simulink model "Mooventure2016_Rev5"  (Simulink 7.7)
settings: Solver=FixedStepDiscrete  StartTime=0.0  StopTime=10  RelTol=1e-3
PreLoadFcn:
  | try, eval([bdroot '_setup']); catch, eval('model_setup', ''); end
InitFcn:
  | try, eval([bdroot '_setup']); catch, eval('model_setup', ''); end
undefined symbols (not defined in the file): ECM, H1, motohawk_build_version, motohawk_trunc_name, motohawk_vardec_config_group, motohawk_vardec_path, xD
libraries: MotoHawk_lib x976, motohawk_control_primitives_lib x41, simulink x27, motohawk_annotations_lib x3
(part 9 of 16)

== system Mooventure2016_Rev5/Foreground/Control/Hybrid Control Code/EcoMode ==
  note: This is brake pedal regen mode
  Inputs : Inport
  InReverse : Inport  Port=2
  Action Port : ActionPort  ActionType=case
  Brake Pedal Scaling : Stateflow chart  TreatAsAtomicUnit=on
  Bus Selector : BusSelector  OutputSignals=Driver Inputs.Throttle_Position (signal 5),Driver Inputs.Brake_Position (signal 2)
  Bus Selector1 : BusSelector  OutputSignals=IPT.ID 260 IPT Status 2.IPT_MotorSpeed
  Chart : Stateflow chart  TreatAsAtomicUnit=on
  Constant : Constant
  Data Type Conversion : DataTypeConversion  OutDataTypeStr=double
  Data Type Conversion1 : DataTypeConversion  OutDataTypeStr=double
  Gas Pedal Scaling : Stateflow chart  TreatAsAtomicUnit=on
  Product : Product  RndMeth=Zero
  Product1 : Product  RndMeth=Zero
  Product2 : Product  RndMeth=Zero
  Sum : Sum
  motohawk_calibration : MotoHawk_lib/Calibration & Probing Blocks/motohawk_calibration  nam='accelStart_Pedal_ecoMode'  val=.02  storage=Calibration  show_more=off  name_source=Use Parameter  data_type=Inherit from 'Default Value'  read_level=1  write_level=1  ovr_cals=on  view_as=Number  enum_struct={'Disabled', 'Enabled'}  vector_style=Wide Row  use_help_units=off  help=''  units=''  use_header_enum=off  row_header_enum={}  col_header_enum={}  use_min_max=off  min_val=-inf  max_val=inf  use_precision=off  precision=''  gain=1  offset=0  exp=1  use_mototune_group=off  mototune_group=motohawk_vardec_path(gcb)
  motohawk_calibration1 : MotoHawk_lib/Calibration & Probing Blocks/motohawk_calibration  nam='brakeStart_Pedal_ecoMode'  val=.02  storage=Calibration  show_more=off  name_source=Use Parameter  data_type=Inherit from 'Default Value'  read_level=1  write_level=1  ovr_cals=on  view_as=Number  enum_struct={'Disabled', 'Enabled'}  vector_style=Wide Row  use_help_units=off  help=''  units=''  use_header_enum=off  row_header_enum={}  col_header_enum={}  use_min_max=off  min_val=-inf  max_val=inf  use_precision=off  precision=''  gain=1  offset=0  exp=1  use_mototune_group=off  mototune_group=motohawk_vardec_path(gcb)
  motohawk_calibration2 : MotoHawk_lib/Calibration & Probing Blocks/motohawk_calibration  nam='brakeEnd_Pedal_ecoMode'  val=.01  storage=Calibration  show_more=off  name_source=Use Parameter  data_type=Inherit from 'Default Value'  read_level=1  write_level=1  ovr_cals=on  view_as=Number  enum_struct={'Disabled', 'Enabled'}  vector_style=Wide Row  use_help_units=off  help=''  units=''  use_header_enum=off  row_header_enum={}  col_header_enum={}  use_min_max=off  min_val=-inf  max_val=inf  use_precision=off  precision=''  gain=1  offset=0  exp=1  use_mototune_group=off  mototune_group=motohawk_vardec_path(gcb)
  motohawk_calibration3 : MotoHawk_lib/Calibration & Probing Blocks/motohawk_calibration  nam='regenStart_Speed_ecoMode'  val=2  storage=Calibration  show_more=off  name_source=Use Parameter  data_type=Inherit from 'Default Value'  read_level=1  write_level=1  ovr_cals=on  view_as=Number  enum_struct={'Disabled', 'Enabled'}  vector_style=Wide Row  use_help_units=off  help=''  units=''  use_header_enum=off  row_header_enum={}  col_header_enum={}  use_min_max=off  min_val=-inf  max_val=inf  use_precision=off  precision=''  gain=1  offset=0  exp=1  use_mototune_group=off  mototune_group=motohawk_vardec_path(gcb)
  motohawk_calibration4 : MotoHawk_lib/Calibration & Probing Blocks/motohawk_calibration  nam='accelEnd_Pedal_ecoMode'  val=.01  storage=Calibration  show_more=off  name_source=Use Parameter  data_type=Inherit from 'Default Value'  read_level=1  write_level=1  ovr_cals=on  view_as=Number  enum_struct={'Disabled', 'Enabled'}  vector_style=Wide Row  use_help_units=off  help=''  units=''  use_header_enum=off  row_header_enum={}  col_header_enum={}  use_min_max=off  min_val=-inf  max_val=inf  use_precision=off  precision=''  gain=1  offset=0  exp=1  use_mototune_group=off  mototune_group=motohawk_vardec_path(gcb)
  motohawk_calibration5 : MotoHawk_lib/Calibration & Probing Blocks/motohawk_calibration  nam='regenEnd_Speed_ecoMode'  val=0.75  storage=Calibration  show_more=off  name_source=Use Parameter  data_type=Inherit from 'Default Value'  read_level=1  write_level=1  ovr_cals=on  view_as=Number  enum_struct={'Disabled', 'Enabled'}  vector_style=Wide Row  use_help_units=off  help=''  units=''  use_header_enum=off  row_header_enum={}  col_header_enum={}  use_min_max=off  min_val=-inf  max_val=inf  use_precision=off  precision=''  gain=1  offset=0  exp=1  use_mototune_group=off  mototune_group=motohawk_vardec_path(gcb)
  motohawk_calibration6 : MotoHawk_lib/Calibration & Probing Blocks/motohawk_calibration  nam='dragTorque_ecoMode'  val=.09  storage=Calibration  show_more=off  name_source=Use Parameter  data_type=Inherit from 'Default Value'  read_level=1  write_level=1  ovr_cals=on  view_as=Number  enum_struct={'Disabled', 'Enabled'}  vector_style=Wide Row  use_help_units=off  help=''  units=''  use_header_enum=off  row_header_enum={}  col_header_enum={}  use_min_max=off  min_val=-inf  max_val=inf  use_precision=off  precision=''  gain=1  offset=0  exp=1  use_mototune_group=off  mototune_group=motohawk_vardec_path(gcb)
  motohawk_calibration7 : MotoHawk_lib/Calibration & Probing Blocks/motohawk_calibration  nam='RPM_to_Wheel_Speed_Multiplier_ecoMode'  val=0.01001896  storage=Calibration  show_more=off  name_source=Use Parameter  data_type=Inherit from 'Default Value'  read_level=1  write_level=1  ovr_cals=on  view_as=Number  enum_struct={'Disabled', 'Enabled'}  vector_style=Wide Row  use_help_units=off  help=''  units=''  use_header_enum=off  row_header_enum={}  col_header_enum={}  use_min_max=off  min_val=-inf  max_val=inf  use_precision=off  precision=''  gain=1  offset=0  exp=1  use_mototune_group=off  mototune_group=motohawk_vardec_path(gcb)
  motohawk_calibration8 : MotoHawk_lib/Calibration & Probing Blocks/motohawk_calibration  nam='driveMaxTorque_ecoMode'  val=1600  storage=Calibration  show_more=off  name_source=Use Parameter  data_type=Inherit from 'Default Value'  read_level=1  write_level=1  ovr_cals=on  view_as=Number  enum_struct={'Disabled', 'Enabled'}  vector_style=Wide Row  use_help_units=off  help=''  units=''  use_header_enum=off  row_header_enum={}  col_header_enum={}  use_min_max=off  min_val=-inf  max_val=inf  use_precision=off  precision=''  gain=1  offset=0  exp=1  use_mototune_group=off  mototune_group=motohawk_vardec_path(gcb)
  motohawk_calibration9 : MotoHawk_lib/Calibration & Probing Blocks/motohawk_calibration  nam='regenMaxTorque_ecoMode'  val=-1500  storage=Calibration  show_more=off  name_source=Use Parameter  data_type=Inherit from 'Default Value'  read_level=1  write_level=1  ovr_cals=on  view_as=Number  enum_struct={'Disabled', 'Enabled'}  vector_style=Wide Row  use_help_units=off  help=''  units=''  use_header_enum=off  row_header_enum={}  col_header_enum={}  use_min_max=off  min_val=-inf  max_val=inf  use_precision=off  precision=''  gain=1  offset=0  exp=1  use_mototune_group=off  mototune_group=motohawk_vardec_path(gcb)
  motohawk_interpolation_1d : MotoHawk_lib/Lookup Tables/motohawk_interpolation_1d  nam='EcoMode_Accel_Map'  table_data=[0:0.05:1]  show_more=on  data_type=double  storage=NonAdaptive  read_level=1  write_level=1  ovr_cals=on  use_help=off  help=''  units=''  use_min_max=off  min_val=0  max_val=1  use_precision=off  precision='1.2'  gain=1  offset=0  exp=1  use_links=on  prelookup_block='EcoMode_Accel'  output_name=''  use_mototune_group=off  mototune_group=motohawk_vardec_path(gcb)
  motohawk_interpolation_1d1 : MotoHawk_lib/Lookup Tables/motohawk_interpolation_1d  nam='EcoMode_Brake_Map'  table_data=[0:0.1:1,1,1,1,1,1,1,1,1,1,1]  show_more=on  data_type=double  storage=NonAdaptive  read_level=1  write_level=1  ovr_cals=on  use_help=off  help=''  units=''  use_min_max=off  min_val=0  max_val=1  use_precision=off  precision='1.2'  gain=1  offset=0  exp=1  use_links=on  prelookup_block='EcoMode_Brake'  output_name=''  use_mototune_group=off  mototune_group=motohawk_vardec_path(gcb)
  motohawk_prelookup : MotoHawk_lib/Lookup Tables/motohawk_prelookup  nam='EcoMode_Accel'  breakpoint_data=[0:0.05:1]  show_more=on  data_type=double  storage=Constant  read_level=1  write_level=1  ovr_cals=on  use_help=off  help=''  units=''  use_min_max=off  min_val=-inf  max_val=inf  use_precision=off  precision=''  gain=1  offset=0  exp=1  use_links=off  input_name=''  use_mototune_group=off  mototune_group=motohawk_vardec_path(gcb)
  motohawk_prelookup1 : MotoHawk_lib/Lookup Tables/motohawk_prelookup  nam='EcoMode_Brake'  breakpoint_data=[0:0.05:1]  show_more=on  data_type=double  storage=Constant  read_level=1  write_level=1  ovr_cals=on  use_help=off  help=''  units=''  use_min_max=off  min_val=-inf  max_val=inf  use_precision=off  precision=''  gain=1  offset=0  exp=1  use_links=off  input_name=''  use_mototune_group=off  mototune_group=motohawk_vardec_path(gcb)
  motohawk_probe : MotoHawk_lib/Calibration & Probing Blocks/motohawk_probe  nam='Gas_Pedal_Prb_EcoMode'  show_more=off  name_source=Use Parameter  read_level=1  view_as=Number  enum_struct={'Disabled', 'Enabled'}  vector_style=Wide Row  use_help_units=off  help=''  units=''  use_header_enum=off  row_header_enum={}  col_header_enum={}  use_precision=off  precision=''  gain=1  offset=0  exp=1  use_mototune_group=off  mototune_group=motohawk_vardec_path(gcb)
  motohawk_probe1 : MotoHawk_lib/Calibration & Probing Blocks/motohawk_probe  nam='driveTorque_Prb_ecoMode'  show_more=off  name_source=Use Parameter  read_level=1  view_as=Number  enum_struct={'Disabled', 'Enabled'}  vector_style=Wide Row  use_help_units=off  help=''  units=''  use_header_enum=off  row_header_enum={}  col_header_enum={}  use_precision=off  precision=''  gain=1  offset=0  exp=1  use_mototune_group=off  mototune_group=motohawk_vardec_path(gcb)
  motohawk_probe2 : MotoHawk_lib/Calibration & Probing Blocks/motohawk_probe  nam='Brake_Pedal_Prb_EcoMode'  show_more=off  name_source=Use Parameter  read_level=1  view_as=Number  enum_struct={'Disabled', 'Enabled'}  vector_style=Wide Row  use_help_units=off  help=''  units=''  use_header_enum=off  row_header_enum={}  col_header_enum={}  use_precision=off  precision=''  gain=1  offset=0  exp=1  use_mototune_group=off  mototune_group=motohawk_vardec_path(gcb)
  motohawk_probe3 : MotoHawk_lib/Calibration & Probing Blocks/motohawk_probe  nam='regenTorque_Prb_ecoMode'  show_more=off  name_source=Use Parameter  read_level=1  view_as=Number  enum_struct={'Disabled', 'Enabled'}  vector_style=Wide Row  use_help_units=off  help=''  units=''  use_header_enum=off  row_header_enum={}  col_header_enum={}  use_precision=off  precision=''  gain=1  offset=0  exp=1  use_mototune_group=off  mototune_group=motohawk_vardec_path(gcb)
  Motor Torque : Outport  InitialOutput=0
  Motor Enable : Outport  Port=2  InitialOutput=0
  wires:
  Inputs/1 -> Bus Selector/1, Bus Selector1/1
  Bus Selector/1 -> Data Type Conversion/1  "<Throttle_Position (signal 5)>"
  Constant/1 -> Motor Enable/1
  Data Type Conversion/1 -> Gas Pedal Scaling/1(throttleIn)  "motor_Torque"
  Gas Pedal Scaling/1(throttleOut) -> motohawk_probe/1, motohawk_prelookup/1  "motor_Torque"
  Data Type Conversion1/1 -> Brake Pedal Scaling/1(brakeIn)
  Brake Pedal Scaling/1(brakeOut) -> motohawk_probe2/1, motohawk_prelookup1/1  "Brake_Pedal"
  InReverse/1 -> Brake Pedal Scaling/2(inReverse)
  Bus Selector/2 -> Data Type Conversion1/1  "<Brake_Position (signal 2)>"
  motohawk_prelookup/1 -> motohawk_interpolation_1d/1
  motohawk_prelookup1/1 -> motohawk_interpolation_1d1/1
  Bus Selector1/1 -> Product/2  "<IPT_MotorSpeed>"
  motohawk_calibration7/1 -> Product/1
  motohawk_interpolation_1d/1 -> Chart/1(accel)
  motohawk_interpolation_1d1/1 -> Chart/2(brake)
  Product/1 -> Chart/3(speed)
  motohawk_calibration/1 -> Chart/4(accelStart)
  motohawk_calibration4/1 -> Chart/5(accelEnd)
  motohawk_calibration1/1 -> Chart/6(brakeStart)
  motohawk_calibration2/1 -> Chart/7(brakeEnd)
  motohawk_calibration3/1 -> Chart/8(regenStart)
  motohawk_calibration5/1 -> Chart/9(regenEnd)
  motohawk_calibration6/1 -> Chart/10(dragTorque)
  Chart/1(driveTorque) -> Product1/1, motohawk_probe1/1
  Chart/2(regenTorque) -> Product2/1, motohawk_probe3/1
  Product1/1 -> Sum/1
  Product2/1 -> Sum/2
  Sum/1 -> Motor Torque/1
  motohawk_calibration8/1 -> Product1/2
  motohawk_calibration9/1 -> Product2/2

== system Mooventure2016_Rev5/Foreground/Control/Hybrid Control Code/Hybrid state limits1 ==
  note: This will put the car into mode 0, disbling all torque
  Inputs : Inport
  Bus Creator : BusCreator  Inputs=2
  Bus Selector : BusSelector  OutputSignals=Driver Inputs.ecoMode (signal 7),Battery_Inputs.StateOfCharge
  Embedded MATLAB Function : Subsystem  TreatAsAtomicUnit=on
  Logical Operator5 : Logic  Operator=NOT  AllPortsSameDT=off  OutDataTypeStr=boolean
  motohawk_calibration1 : MotoHawk_lib/Calibration & Probing Blocks/motohawk_calibration  nam='CrawlHomeEnterSOC'  val=14  storage=Calibration  show_more=on  name_source=Use Parameter  data_type=Inherit from 'Default Value'  read_level=1  write_level=1  ovr_cals=on  view_as=Number  enum_struct={'Disabled', 'Enabled'}  vector_style=Wide Row  use_help_units=on  help='Minimum SOC to assist'  units='%'  use_header_enum=off  row_header_enum={}  col_header_enum={}  use_min_max=on  min_val=0  max_val=100  use_precision=off  precision=''  gain=1  offset=0  exp=1  use_mototune_group=off  mototune_group=motohawk_vardec_path(gcb)
  motohawk_calibration2 : MotoHawk_lib/Calibration & Probing Blocks/motohawk_calibration  nam='SafetyModeEnterSOC'  val=5  storage=Calibration  show_more=on  name_source=Use Parameter  data_type=Inherit from 'Default Value'  read_level=1  write_level=1  ovr_cals=on  view_as=Number  enum_struct={'Disabled', 'Enabled'}  vector_style=Wide Row  use_help_units=on  help='Minimum SOC to assist'  units='%'  use_header_enum=off  row_header_enum={}  col_header_enum={}  use_min_max=on  min_val=0  max_val=100  use_precision=off  precision=''  gain=1  offset=0  exp=1  use_mototune_group=off  mototune_group=motohawk_vardec_path(gcb)
  motohawk_data_read : MotoHawk_lib/Data Storage Blocks/motohawk_data_read  source=Lookup By Name  structure=Scalar  operation=Read scalar from location by index  sz_vec=4  sz_row=2  sz_col=3  typ=boolean  nam='Torque_Enable'  checkNull=on  struct_inst_name='MyData'  struct_nam='MyStruct'
  state_o : Outport
  SoCBounds : Outport  Port=2
  wires:
  Embedded MATLAB Function/1(state) -> state_o/1
  Logical Operator5/1 -> Embedded MATLAB Function/5(nEV)
  Inputs/1 -> Bus Selector/1
  Bus Selector/1 -> Embedded MATLAB Function/1(ecoMode_Enable)  "<ecoMode (signal 7)>"
  Bus Selector/2 -> Embedded MATLAB Function/2(SOC)  "<StateOfCharge>"
  motohawk_calibration2/1 -> Bus Creator/2, Embedded MATLAB Function/4(SMESoC)  "SafetyModeBoundSoC"
  Bus Creator/1 -> SoCBounds/1
  motohawk_calibration1/1 -> Bus Creator/1, Embedded MATLAB Function/3(CHESoC)  "CrawlHomeBoundSoC"
  motohawk_data_read/1 -> Logical Operator5/1

== system Mooventure2016_Rev5/Foreground/Control/Hybrid Control Code/IPT ==
  note: 1 - reverse
      | 2 - neutral
      | 3 - drive
  note: Merge does addition
  note: Filter to remove "debouncing" noise from the line.
      |
      | Whenever we have a signal, we have noise that can be interpreted "too well" where
      | tiny fluctuations cause changes we don't want to experience in a car.
      | Putting it through a filter will "smooth out" this noise.
  note: Saturation block to limit max and min torque values
  note: This will limit performance of motor if necessary
  note: Thse bottom 3 subsystems multiply the torque be 1,0,-1 in order to
      | send torque in the right direction
  In1 : Inport
  In2 : Inport  Port=2
  Bus Selector : BusSelector  OutputSignals=Battery_Inputs.BatteryCurrent,Driver Inputs.Shift_Position (signal 4)
  Compare To Constant : simulink/Logic and Bit Operations/Compare To Constant  SystemSampleTime=-1  relop===  const=2  LogicOutDataTypeMode=boolean
  Compare To Constant1 : simulink/Logic and Bit Operations/Compare To Constant  SystemSampleTime=-1  relop===  const=3  LogicOutDataTypeMode=boolean
  Compare To Constant2 : simulink/Logic and Bit Operations/Compare To Constant  SystemSampleTime=-1  relop===  const=1  LogicOutDataTypeMode=boolean
  Constant1 : Constant
  CurrentLimiting_TurboRequest : Subsystem
  Drive : Subsystem  TreatAsAtomicUnit=on
  First Order Low Pass (Tunable) : Subsystem  mask(First-Order Low-Pass Filter (Tunable)){nam='FiltConst', samp_time=-1, group=motohawk_vardec_path(gcb)}
      mask prompts: nam "Name"; samp_time "Sample Time"; group "MotoTune Group String"
      mask help:
      | Discrete first-order low-pass filter, with calibratable time-constant.
      |
      | If 'Sample Time' is -1, then extra code and RAM will be generated to dynamically calculate dt.
      mask Display:
      | patch([0 0 1 1], [0 0.075 0.075 0], [230/255 0/255 0/255])
      | patch([0 0 1 1], [0.025 0.05 0.05 0.025], [150/255 0/255 0/255])
      | patch([0 0 1 1], [0 0.025 0.025 0], [0/255 0/255 0/255])
      | 
      | disp('1st-Order\nLow Pass');
  Merge : Merge  Inputs=3
  Neutral : Subsystem  TreatAsAtomicUnit=on
  Product : Product  Inputs=3  RndMeth=Zero
  Reverse : Subsystem  TreatAsAtomicUnit=on
  Saturation : Saturate  UpperLimit=2500  LowerLimit=-2500
  Switch1 : Switch  Criteria=u2 ~= 0
  motohawk_calibration1 : MotoHawk_lib/Calibration & Probing Blocks/motohawk_calibration  nam='CurrentLimitingEnabled'  val=0  storage=Calibration  show_more=off  name_source=Use Parameter  data_type=Inherit from 'Default Value'  read_level=1  write_level=1  ovr_cals=on  view_as=Number  enum_struct={'Disabled', 'Enabled'}  vector_style=Wide Row  use_help_units=off  help=''  units=''  use_header_enum=off  row_header_enum={}  col_header_enum={}  use_min_max=off  min_val=-inf  max_val=inf  use_precision=off  precision=''  gain=1  offset=0  exp=1  use_mototune_group=off  mototune_group=motohawk_vardec_path(gcb)
  motohawk_override_abs : MotoHawk_lib/Calibration & Probing Blocks/motohawk_override_abs  SystemSampleTime=-1  parent_name='Torque_Request_Override'  parent_val=0  show_more=off  name_source=Use Parameter  parent_read_level=1  parent_override_level=1  view_as=Number  enum_struct={'Disabled', 'Enabled'}  use_help_units=off  parent_help=''  parent_units=''  use_min_max=off  parent_min=-inf  parent_max=inf  use_precision=off  parent_precision=''  parent_gain=1  parent_offset=0  parent_exp=1  use_mototune_group=off  parent_group=motohawk_vardec_path(gcb)
  motohawk_probe1 : MotoHawk_lib/Calibration & Probing Blocks/motohawk_probe  nam='Torque_Request_Probe'  show_more=off  name_source=Use Parameter  read_level=1  view_as=Number  enum_struct={'Disabled', 'Enabled'}  vector_style=Wide Row  use_help_units=off  help=''  units=''  use_header_enum=off  row_header_enum={}  col_header_enum={}  use_precision=off  precision=''  gain=1  offset=0  exp=1  use_mototune_group=off  mototune_group=motohawk_vardec_path(gcb)
  motohawk_probe3 : MotoHawk_lib/Calibration & Probing Blocks/motohawk_probe  nam='IPT_Direction_Prb'  show_more=off  name_source=Use Parameter  read_level=1  view_as=Number  enum_struct={'Disabled', 'Enabled'}  vector_style=Wide Row  use_help_units=off  help=''  units=''  use_header_enum=off  row_header_enum={}  col_header_enum={}  use_precision=off  precision=''  gain=1  offset=0  exp=1  use_mototune_group=off  mototune_group=motohawk_vardec_path(gcb)
  motohawk_probe4 : MotoHawk_lib/Calibration & Probing Blocks/motohawk_probe  nam='pre_Filter_Torque_Request'  show_more=off  name_source=Use Parameter  read_level=1  view_as=Number  enum_struct={'Disabled', 'Enabled'}  vector_style=Wide Row  use_help_units=off  help=''  units=''  use_header_enum=off  row_header_enum={}  col_header_enum={}  use_precision=off  precision=''  gain=1  offset=0  exp=1  use_mototune_group=off  mototune_group=motohawk_vardec_path(gcb)
  Torque_Request : Outport  OutputWhenDisabled=reset  InitialOutput=[0]
  IPT_Direction : Outport  Port=2  OutputWhenDisabled=reset  InitialOutput=[0]
  InReverse : Outport  Port=3
  wires:
  Compare To Constant2/1 -> Reverse/Enable, InReverse/1
  Compare To Constant1/1 -> Drive/Enable
  Neutral/1(IPT_Torque) -> Merge/1
  Product/1 -> First Order Low Pass (Tunable)/1(in), motohawk_probe4/1  "IPT_Torque_Request"
  First Order Low Pass (Tunable)/1(out) -> Saturation/1  "Torque_Request"
  Bus Selector/2 -> Compare To Constant/1, Compare To Constant2/1, Compare To Constant1/1  "<Shift_Position (signal 4)>"
  motohawk_calibration1/1 -> Switch1/2
  Constant1/1 -> Switch1/3
  CurrentLimiting_TurboRequest/1(TorqueMultiplier) -> Switch1/1
  Switch1/1 -> Product/1
  In1/1 -> Bus Selector/1  "Inputs"
  Bus Selector/1 -> CurrentLimiting_TurboRequest/1(BatteryCurrent)  "<BatteryCurrent>"
  Drive/1(IPT_Torque) -> Merge/2
  Reverse/1(IPT_Torque) -> Merge/3
  motohawk_override_abs/1 -> Torque_Request/1  "Torque_Request"
  Compare To Constant/1 -> Neutral/Enable
  Saturation/1 -> motohawk_override_abs/1, motohawk_probe1/1
  Merge/1 -> Product/2, IPT_Direction/1, motohawk_probe3/1  "Torque_Direction"
  In2/1 -> Product/3  "TorqueRequest"

== system Mooventure2016_Rev5/Foreground/Control/Hybrid Control Code/SUVMode ==
  note: This is brake pedal regen mode
  Inputs : Inport
  InReverse : Inport  Port=2
  Action Port : ActionPort  ActionType=case
  Brake Pedal Scaling : Stateflow chart  TreatAsAtomicUnit=on
  Bus Selector : BusSelector  OutputSignals=Driver Inputs.Throttle_Position (signal 5),Driver Inputs.Brake_Position (signal 2)
  Bus Selector1 : BusSelector  OutputSignals=IPT.ID 260 IPT Status 2.IPT_MotorSpeed
  Chart : Stateflow chart  TreatAsAtomicUnit=on
  Constant : Constant
  Data Type Conversion : DataTypeConversion  OutDataTypeStr=double
  Data Type Conversion1 : DataTypeConversion  OutDataTypeStr=double
  Gas Pedal Scaling : Stateflow chart  TreatAsAtomicUnit=on
  Product : Product  RndMeth=Zero
  Product1 : Product  RndMeth=Zero
  Product2 : Product  RndMeth=Zero
  Sum : Sum
  motohawk_calibration : MotoHawk_lib/Calibration & Probing Blocks/motohawk_calibration  nam='accelStart_Pedal_SUVMode'  val=.02  storage=Calibration  show_more=on  name_source=Use Parameter  data_type=Inherit from 'Default Value'  read_level=1  write_level=1  ovr_cals=on  view_as=Number  enum_struct={'Disabled', 'Enabled'}  vector_style=Wide Row  use_help_units=on  help=''  units='%'  use_header_enum=off  row_header_enum={}  col_header_enum={}  use_min_max=off  min_val=-inf  max_val=inf  use_precision=off  precision=''  gain=1  offset=0  exp=1  use_mototune_group=off  mototune_group=motohawk_vardec_path(gcb)
  motohawk_calibration1 : MotoHawk_lib/Calibration & Probing Blocks/motohawk_calibration  nam='brakeStart_Pedal_SUVMode'  val=.02  storage=Calibration  show_more=off  name_source=Use Parameter  data_type=Inherit from 'Default Value'  read_level=1  write_level=1  ovr_cals=on  view_as=Number  enum_struct={'Disabled', 'Enabled'}  vector_style=Wide Row  use_help_units=off  help=''  units=''  use_header_enum=off  row_header_enum={}  col_header_enum={}  use_min_max=off  min_val=-inf  max_val=inf  use_precision=off  precision=''  gain=1  offset=0  exp=1  use_mototune_group=off  mototune_group=motohawk_vardec_path(gcb)
  motohawk_calibration2 : MotoHawk_lib/Calibration & Probing Blocks/motohawk_calibration  nam='brakeEnd_Pedal_SUVMode'  val=.01  storage=Calibration  show_more=off  name_source=Use Parameter  data_type=Inherit from 'Default Value'  read_level=1  write_level=1  ovr_cals=on  view_as=Number  enum_struct={'Disabled', 'Enabled'}  vector_style=Wide Row  use_help_units=off  help=''  units=''  use_header_enum=off  row_header_enum={}  col_header_enum={}  use_min_max=off  min_val=-inf  max_val=inf  use_precision=off  precision=''  gain=1  offset=0  exp=1  use_mototune_group=off  mototune_group=motohawk_vardec_path(gcb)
  motohawk_calibration3 : MotoHawk_lib/Calibration & Probing Blocks/motohawk_calibration  nam='regenStart_Speed_SUVMode'  val=2  storage=Calibration  show_more=off  name_source=Use Parameter  data_type=Inherit from 'Default Value'  read_level=1  write_level=1  ovr_cals=on  view_as=Number  enum_struct={'Disabled', 'Enabled'}  vector_style=Wide Row  use_help_units=off  help=''  units=''  use_header_enum=off  row_header_enum={}  col_header_enum={}  use_min_max=off  min_val=-inf  max_val=inf  use_precision=off  precision=''  gain=1  offset=0  exp=1  use_mototune_group=off  mototune_group=motohawk_vardec_path(gcb)
  motohawk_calibration4 : MotoHawk_lib/Calibration & Probing Blocks/motohawk_calibration  nam='accelEnd_Pedal_SUVMode'  val=.01  storage=Calibration  show_more=off  name_source=Use Parameter  data_type=Inherit from 'Default Value'  read_level=1  write_level=1  ovr_cals=on  view_as=Number  enum_struct={'Disabled', 'Enabled'}  vector_style=Wide Row  use_help_units=off  help=''  units=''  use_header_enum=off  row_header_enum={}  col_header_enum={}  use_min_max=off  min_val=-inf  max_val=inf  use_precision=off  precision=''  gain=1  offset=0  exp=1  use_mototune_group=off  mototune_group=motohawk_vardec_path(gcb)
  motohawk_calibration5 : MotoHawk_lib/Calibration & Probing Blocks/motohawk_calibration  nam='regenEnd_Speed_SUVMode'  val=0.75  storage=Calibration  show_more=off  name_source=Use Parameter  data_type=Inherit from 'Default Value'  read_level=1  write_level=1  ovr_cals=on  view_as=Number  enum_struct={'Disabled', 'Enabled'}  vector_style=Wide Row  use_help_units=off  help=''  units=''  use_header_enum=off  row_header_enum={}  col_header_enum={}  use_min_max=off  min_val=-inf  max_val=inf  use_precision=off  precision=''  gain=1  offset=0  exp=1  use_mototune_group=off  mototune_group=motohawk_vardec_path(gcb)
  motohawk_calibration6 : MotoHawk_lib/Calibration & Probing Blocks/motohawk_calibration  nam='dragTorque_SUVMode'  val=.095  storage=Calibration  show_more=off  name_source=Use Parameter  data_type=Inherit from 'Default Value'  read_level=1  write_level=1  ovr_cals=on  view_as=Number  enum_struct={'Disabled', 'Enabled'}  vector_style=Wide Row  use_help_units=off  help=''  units=''  use_header_enum=off  row_header_enum={}  col_header_enum={}  use_min_max=off  min_val=-inf  max_val=inf  use_precision=off  precision=''  gain=1  offset=0  exp=1  use_mototune_group=off  mototune_group=motohawk_vardec_path(gcb)
  motohawk_calibration7 : MotoHawk_lib/Calibration & Probing Blocks/motohawk_calibration  nam='RPM_to_Wheel_Speed_Multiplier_SUVMode'  val=0.01001896  storage=Calibration  show_more=off  name_source=Use Parameter  data_type=Inherit from 'Default Value'  read_level=1  write_level=1  ovr_cals=on  view_as=Number  enum_struct={'Disabled', 'Enabled'}  vector_style=Wide Row  use_help_units=off  help=''  units=''  use_header_enum=off  row_header_enum={}  col_header_enum={}  use_min_max=off  min_val=-inf  max_val=inf  use_precision=off  precision=''  gain=1  offset=0  exp=1  use_mototune_group=off  mototune_group=motohawk_vardec_path(gcb)
  motohawk_calibration8 : MotoHawk_lib/Calibration & Probing Blocks/motohawk_calibration  nam='driveMaxTorque_SUVMode'  val=2500  storage=Calibration  show_more=off  name_source=Use Parameter  data_type=Inherit from 'Default Value'  read_level=1  write_level=1  ovr_cals=on  view_as=Number  enum_struct={'Disabled', 'Enabled'}  vector_style=Wide Row  use_help_units=off  help=''  units=''  use_header_enum=off  row_header_enum={}  col_header_enum={}  use_min_max=off  min_val=-inf  max_val=inf  use_precision=off  precision=''  gain=1  offset=0  exp=1  use_mototune_group=off  mototune_group=motohawk_vardec_path(gcb)
  motohawk_calibration9 : MotoHawk_lib/Calibration & Probing Blocks/motohawk_calibration  nam='regenMaxTorque_SUVMode'  val=-1500  storage=Calibration  show_more=off  name_source=Use Parameter  data_type=Inherit from 'Default Value'  read_level=1  write_level=1  ovr_cals=on  view_as=Number  enum_struct={'Disabled', 'Enabled'}  vector_style=Wide Row  use_help_units=off  help=''  units=''  use_header_enum=off  row_header_enum={}  col_header_enum={}  use_min_max=off  min_val=-inf  max_val=inf  use_precision=off  precision=''  gain=1  offset=0  exp=1  use_mototune_group=off  mototune_group=motohawk_vardec_path(gcb)
  motohawk_interpolation_1d : MotoHawk_lib/Lookup Tables/motohawk_interpolation_1d  nam='SUVMode_Accel_Map'  table_data=[0,0.05,0.1,0.15,0.2,0.3,0.4,0.5,0.6,0.7,0.8,0.9,1,1,1,1,1,1,1,1,1]  show_more=on  data_type=double  storage=NonAdaptive  read_level=1  write_level=1  ovr_cals=on  use_help=off  help=''  units=''  use_min_max=off  min_val=0  max_val=1  use_precision=off  precision='1.2'  gain=1  offset=0  exp=1  use_links=on  prelookup_block='SUVMode_Accel'  output_name=''  use_mototune_group=off  mototune_group=motohawk_vardec_path(gcb)
  motohawk_interpolation_1d1 : MotoHawk_lib/Lookup Tables/motohawk_interpolation_1d  nam='SUVMode_Brake_Map'  table_data=[0:0.1:1,1,1,1,1,1,1,1,1,1,1]  show_more=on  data_type=double  storage=NonAdaptive  read_level=1  write_level=1  ovr_cals=on  use_help=off  help=''  units=''  use_min_max=off  min_val=0  max_val=1  use_precision=off  precision='1.2'  gain=1  offset=0  exp=1  use_links=on  prelookup_block='SUVMode_Brake'  output_name=''  use_mototune_group=off  mototune_group=motohawk_vardec_path(gcb)
  motohawk_prelookup : MotoHawk_lib/Lookup Tables/motohawk_prelookup  nam='SUVMode_Accel'  breakpoint_data=[0:0.05:1]  show_more=on  data_type=double  storage=Constant  read_level=1  write_level=1  ovr_cals=on  use_help=off  help=''  units=''  use_min_max=off  min_val=-inf  max_val=inf  use_precision=off  precision=''  gain=1  offset=0  exp=1  use_links=off  input_name=''  use_mototune_group=off  mototune_group=motohawk_vardec_path(gcb)
  motohawk_prelookup1 : MotoHawk_lib/Lookup Tables/motohawk_prelookup  nam='SUVMode_Brake'  breakpoint_data=[0:0.05:1]  show_more=on  data_type=double  storage=Constant  read_level=1  write_level=1  ovr_cals=on  use_help=off  help=''  units=''  use_min_max=off  min_val=-inf  max_val=inf  use_precision=off  precision=''  gain=1  offset=0  exp=1  use_links=off  input_name=''  use_mototune_group=off  mototune_group=motohawk_vardec_path(gcb)
  motohawk_probe : MotoHawk_lib/Calibration & Probing Blocks/motohawk_probe  nam='Gas_Pedal_Prb_SUVMode'  show_more=off  name_source=Use Parameter  read_level=1  view_as=Number  enum_struct={'Disabled', 'Enabled'}  vector_style=Wide Row  use_help_units=off  help=''  units=''  use_header_enum=off  row_header_enum={}  col_header_enum={}  use_precision=off  precision=''  gain=1  offset=0  exp=1  use_mototune_group=off  mototune_group=motohawk_vardec_path(gcb)
  motohawk_probe1 : MotoHawk_lib/Calibration & Probing Blocks/motohawk_probe  nam='driveTorque_Prb_SUVMode'  show_more=off  name_source=Use Parameter  read_level=1  view_as=Number  enum_struct={'Disabled', 'Enabled'}  vector_style=Wide Row  use_help_units=off  help=''  units=''  use_header_enum=off  row_header_enum={}  col_header_enum={}  use_precision=off  precision=''  gain=1  offset=0  exp=1  use_mototune_group=off  mototune_group=motohawk_vardec_path(gcb)
  motohawk_probe2 : MotoHawk_lib/Calibration & Probing Blocks/motohawk_probe  nam='Brake_Pedal_Prb_SUVMode'  show_more=off  name_source=Use Parameter  read_level=1  view_as=Number  enum_struct={'Disabled', 'Enabled'}  vector_style=Wide Row  use_help_units=off  help=''  units=''  use_header_enum=off  row_header_enum={}  col_header_enum={}  use_precision=off  precision=''  gain=1  offset=0  exp=1  use_mototune_group=off  mototune_group=motohawk_vardec_path(gcb)
  motohawk_probe3 : MotoHawk_lib/Calibration & Probing Blocks/motohawk_probe  nam='regenTorque_Prb_SUVMode'  show_more=off  name_source=Use Parameter  read_level=1  view_as=Number  enum_struct={'Disabled', 'Enabled'}  vector_style=Wide Row  use_help_units=off  help=''  units=''  use_header_enum=off  row_header_enum={}  col_header_enum={}  use_precision=off  precision=''  gain=1  offset=0  exp=1  use_mototune_group=off  mototune_group=motohawk_vardec_path(gcb)
  Motor Torque : Outport  InitialOutput=0
  Motor Enable : Outport  Port=2  InitialOutput=0
  wires:
  Inputs/1 -> Bus Selector/1, Bus Selector1/1
  Bus Selector/1 -> Data Type Conversion/1  "<Throttle_Position (signal 5)>"
  Constant/1 -> Motor Enable/1
  Data Type Conversion/1 -> Gas Pedal Scaling/1(throttleIn)  "motor_Torque"
  Gas Pedal Scaling/1(throttleOut) -> motohawk_probe/1, motohawk_prelookup/1  "motor_Torque"
  Data Type Conversion1/1 -> Brake Pedal Scaling/1(brakeIn)
  Brake Pedal Scaling/1(brakeOut) -> motohawk_probe2/1, motohawk_prelookup1/1  "Brake_Pedal"
  InReverse/1 -> Brake Pedal Scaling/2(inReverse)
  Bus Selector/2 -> Data Type Conversion1/1  "<Brake_Position (signal 2)>"
  motohawk_prelookup/1 -> motohawk_interpolation_1d/1
  motohawk_prelookup1/1 -> motohawk_interpolation_1d1/1
  Bus Selector1/1 -> Product/2  "<IPT_MotorSpeed>"
  motohawk_calibration7/1 -> Product/1
  motohawk_interpolation_1d/1 -> Chart/1(accel)
  motohawk_interpolation_1d1/1 -> Chart/2(brake)
  Product/1 -> Chart/3(speed)
  motohawk_calibration/1 -> Chart/4(accelStart)
  motohawk_calibration4/1 -> Chart/5(accelEnd)
  motohawk_calibration1/1 -> Chart/6(brakeStart)
  motohawk_calibration2/1 -> Chart/7(brakeEnd)
  motohawk_calibration3/1 -> Chart/8(regenStart)
  motohawk_calibration5/1 -> Chart/9(regenEnd)
  motohawk_calibration6/1 -> Chart/10(dragTorque)
  Chart/1(driveTorque) -> Product1/1, motohawk_probe1/1
  Chart/2(regenTorque) -> Product2/1, motohawk_probe3/1
  Product1/1 -> Sum/1
  Product2/1 -> Sum/2
  Sum/1 -> Motor Torque/1
  motohawk_calibration8/1 -> Product1/2
  motohawk_calibration9/1 -> Product2/2

== system Mooventure2016_Rev5/Foreground/Control/Hybrid Control Code/Safety ==
  note: In this mode the motor will not spin and it will not enable,
      | so no DCDC converter, or Heat. Charger should
      | still work though in order to charge car
  Inputs : Inport
  Action Port : ActionPort  ActionType=case
  Constant : Constant  Value=0
  Constant2 : Constant  Value=0
  Terminator : Terminator
  Motor Torque : Outport  InitialOutput=0
  Motor Enable : Outport  Port=2  InitialOutput=0
  wires:
  Constant2/1 -> Motor Enable/1  "motor_Enable"
  Inputs/1 -> Terminator/1
  Constant/1 -> Motor Torque/1  "motor_Torque"

== system Mooventure2016_Rev5/Foreground/Control/Hybrid Control Code/Traction Control ==
  In1 : Inport
  Switch : Switch  Threshold=1
  Torque Limiter : Stateflow chart  TreatAsAtomicUnit=on
  motohawk_calibration : MotoHawk_lib/Calibration & Probing Blocks/motohawk_calibration  nam='Traction_Control_Enable'  val=0  storage=Calibration  show_more=off  name_source=Use Parameter  data_type=Inherit from 'Default Value'  read_level=1  write_level=1  ovr_cals=on  view_as=Number  enum_struct={'Disabled', 'Enabled'}  vector_style=Wide Row  use_help_units=off  help=''  units=''  use_header_enum=off  row_header_enum={}  col_header_enum={}  use_min_max=off  min_val=-inf  max_val=inf  use_precision=off  precision=''  gain=1  offset=0  exp=1  use_mototune_group=off  mototune_group=motohawk_vardec_path(gcb)
  motohawk_calibration1 : MotoHawk_lib/Calibration & Probing Blocks/motohawk_calibration  nam='Traction_Control_Max_Torque'  val=300  storage=Calibration  show_more=off  name_source=Use Parameter  data_type=Inherit from 'Default Value'  read_level=1  write_level=1  ovr_cals=on  view_as=Number  enum_struct={'Disabled', 'Enabled'}  vector_style=Wide Row  use_help_units=off  help=''  units=''  use_header_enum=off  row_header_enum={}  col_header_enum={}  use_min_max=off  min_val=-inf  max_val=inf  use_precision=off  precision=''  gain=1  offset=0  exp=1  use_mototune_group=off  mototune_group=motohawk_vardec_path(gcb)
  Out1 : Outport
  wires:
  In1/1 -> Switch/3, Torque Limiter/2(torqueIn)
  motohawk_calibration/1 -> Switch/2
  Switch/1 -> Out1/1
  Torque Limiter/1(torqueOut) -> Switch/1
  motohawk_calibration1/1 -> Torque Limiter/1(maxTorque)

== system Mooventure2016_Rev5/Foreground/Inputs/Analog Inputs/Contactors ==
  Bus Creator : BusCreator
  motohawk_calibration : MotoHawk_lib/Calibration & Probing Blocks/motohawk_calibration  nam='Contactor1'  val=0  storage=Calibration  show_more=off  name_source=Use Parameter  data_type=Inherit from 'Default Value'  read_level=1  write_level=1  ovr_cals=on  view_as=Number  enum_struct={'Disabled', 'Enabled'}  vector_style=Wide Row  use_help_units=off  help=''  units=''  use_header_enum=off  row_header_enum={}  col_header_enum={}  use_min_max=off  min_val=-inf  max_val=inf  use_precision=off  precision=''  gain=1  offset=0  exp=1  use_mototune_group=off  mototune_group=motohawk_vardec_path(gcb)
  motohawk_calibration1 : MotoHawk_lib/Calibration & Probing Blocks/motohawk_calibration  nam='Contactor2'  val=0  storage=Calibration  show_more=off  name_source=Use Parameter  data_type=Inherit from 'Default Value'  read_level=1  write_level=1  ovr_cals=on  view_as=Number  enum_struct={'Disabled', 'Enabled'}  vector_style=Wide Row  use_help_units=off  help=''  units=''  use_header_enum=off  row_header_enum={}  col_header_enum={}  use_min_max=off  min_val=-inf  max_val=inf  use_precision=off  precision=''  gain=1  offset=0  exp=1  use_mototune_group=off  mototune_group=motohawk_vardec_path(gcb)
  motohawk_calibration2 : MotoHawk_lib/Calibration & Probing Blocks/motohawk_calibration  nam='Contactor3'  val=0  storage=Calibration  show_more=off  name_source=Use Parameter  data_type=Inherit from 'Default Value'  read_level=1  write_level=1  ovr_cals=on  view_as=Number  enum_struct={'Disabled', 'Enabled'}  vector_style=Wide Row  use_help_units=off  help=''  units=''  use_header_enum=off  row_header_enum={}  col_header_enum={}  use_min_max=off  min_val=-inf  max_val=inf  use_precision=off  precision=''  gain=1  offset=0  exp=1  use_mototune_group=off  mototune_group=motohawk_vardec_path(gcb)
  motohawk_calibration3 : MotoHawk_lib/Calibration & Probing Blocks/motohawk_calibration  nam='Contactor4'  val=0  storage=Calibration  show_more=off  name_source=Use Parameter  data_type=Inherit from 'Default Value'  read_level=1  write_level=1  ovr_cals=on  view_as=Number  enum_struct={'Disabled', 'Enabled'}  vector_style=Wide Row  use_help_units=off  help=''  units=''  use_header_enum=off  row_header_enum={}  col_header_enum={}  use_min_max=off  min_val=-inf  max_val=inf  use_precision=off  precision=''  gain=1  offset=0  exp=1  use_mototune_group=off  mototune_group=motohawk_vardec_path(gcb)
  Out1 : Outport
  wires:
  motohawk_calibration3/1 -> Bus Creator/4  "Contactor4"
  motohawk_calibration2/1 -> Bus Creator/3  "Contactor3"
  motohawk_calibration1/1 -> Bus Creator/2  "Contactor2"
  motohawk_calibration/1 -> Bus Creator/1  "Contactor1"
  Bus Creator/1 -> Out1/1

== system Mooventure2016_Rev5/Foreground/Inputs/Analog Inputs/Coolant ==
  Bus Creator : BusCreator
  Data Type Conversion : DataTypeConversion  OutDataTypeStr=double
  Data Type Conversion1 : DataTypeConversion  OutDataTypeStr=double
  Data Type Conversion2 : DataTypeConversion  OutDataTypeStr=double
  Embedded MATLAB Function : Stateflow chart  TreatAsAtomicUnit=on
  Heater Core Low Pass : Subsystem  mask(First-Order Low-Pass Filter (Tunable)){nam='HtrCoreLowPass', samp_time=-1, group=motohawk_vardec_path(gcb)}
      mask prompts: nam "Name"; samp_time "Sample Time"; group "MotoTune Group String"
      mask help:
      | Discrete first-order low-pass filter, with calibratable time-constant.
      |
      | If 'Sample Time' is -1, then extra code and RAM will be generated to dynamically calculate dt.
      mask Display:
      | patch([0 0 1 1], [0 0.075 0.075 0], [230/255 0/255 0/255])
      | patch([0 0 1 1], [0.025 0.05 0.05 0.025], [150/255 0/255 0/255])
      | patch([0 0 1 1], [0 0.025 0.025 0], [0/255 0/255 0/255])
      | 
      | disp('1st-Order\nLow Pass');
  Radiator Low Pass : Subsystem  mask(First-Order Low-Pass Filter (Tunable)){nam='RadLowPass', samp_time=-1, group=motohawk_vardec_path(gcb)}
      mask prompts: nam "Name"; samp_time "Sample Time"; group "MotoTune Group String"
      mask help:
      | Discrete first-order low-pass filter, with calibratable time-constant.
      |
      | If 'Sample Time' is -1, then extra code and RAM will be generated to dynamically calculate dt.
      mask Display:
      | patch([0 0 1 1], [0 0.075 0.075 0], [230/255 0/255 0/255])
      | patch([0 0 1 1], [0.025 0.05 0.05 0.025], [150/255 0/255 0/255])
      | patch([0 0 1 1], [0 0.025 0.025 0], [0/255 0/255 0/255])
      | 
      | disp('1st-Order\nLow Pass');
  Terminator : Terminator
  Terminator1 : Terminator
  Terminator2 : Terminator
  motohawk_ain1 : MotoHawk_lib/Analog I//O Blocks/motohawk_ain  res_name=[]  text_resource=AN14  code_resource=NONE  val_resource=-1  target=ECM-5554-112-0904-xD  resource_enum_str=(None)=-1,AN24=1,AN25=2,AN26=3,AN27=4,AN28=5,AN29=6,AN30=7,AN31=8,AN32=9,AN33=10,ECUP=11,ESTOP=12,DRVP=13,XDRP=14,XDRP_B=15,AN1=16,AN2=17,AN3=18,AN4=19,AN5=20,AN6=21,AN7=22,AN8=23,AN9=24,AN10=25,AN11=26,AN12=27,AN13=28,AN14=29,AN15=30,AN16=31,AN17=32,AN18=33,AN19=34,AN20=35,AN21=36,AN22=37,AN23=38,O2A=39,O2B=40,O2C=41,O2D=42  altref=5V Reference  typ=uint16  num_adc_bits=8  use_stat=on  use_vardec=on  nam='Heater_Core_Blend_Position'  read_level=1  write_level=1  group='I/O Pins | Inputs Config'
  motohawk_ain2 : MotoHawk_lib/Analog I//O Blocks/motohawk_ain  res_name=[]  text_resource=AN2  code_resource=NONE  val_resource=-1  target=ECM-5554-112-0904-xD  resource_enum_str=(None)=-1,AN24=1,AN25=2,AN26=3,AN27=4,AN28=5,AN29=6,AN30=7,AN31=8,AN32=9,AN33=10,ECUP=11,ESTOP=12,DRVP=13,XDRP=14,XDRP_B=15,AN1=16,AN2=17,AN3=18,AN4=19,AN5=20,AN6=21,AN7=22,AN8=23,AN9=24,AN10=25,AN11=26,AN12=27,AN13=28,AN14=29,AN15=30,AN16=31,AN17=32,AN18=33,AN19=34,AN20=35,AN21=36,AN22=37,AN23=38,O2A=39,O2B=40,O2C=41,O2D=42  altref=5V Reference  typ=uint16  num_adc_bits=8  use_stat=on  use_vardec=on  nam='Radiator_Blend_Position'  read_level=1  write_level=1  group='I/O Pins | Inputs Config'
  motohawk_ain4 : MotoHawk_lib/Analog I//O Blocks/motohawk_ain  res_name=[]  text_resource=AN3  code_resource=NONE  val_resource=-1  target=ECM-5554-112-0904-xD  resource_enum_str=(None)=-1,AN24=1,AN25=2,AN26=3,AN27=4,AN28=5,AN29=6,AN30=7,AN31=8,AN32=9,AN33=10,ECUP=11,ESTOP=12,DRVP=13,XDRP=14,XDRP_B=15,AN1=16,AN2=17,AN3=18,AN4=19,AN5=20,AN6=21,AN7=22,AN8=23,AN9=24,AN10=25,AN11=26,AN12=27,AN13=28,AN14=29,AN15=30,AN16=31,AN17=32,AN18=33,AN19=34,AN20=35,AN21=36,AN22=37,AN23=38,O2A=39,O2B=40,O2C=41,O2D=42  altref=5V Reference  typ=uint16  num_adc_bits=8  use_stat=on  use_vardec=on  nam='Heater_Temp'  read_level=1  write_level=1  group='I/O Pins | Inputs Config'
  motohawk_override_abs1 : MotoHawk_lib/Calibration & Probing Blocks/motohawk_override_abs  SystemSampleTime=-1  parent_name='Radiator_Blend_Valve_Ovr'  parent_val=0  show_more=off  name_source=Use Parameter  parent_read_level=1  parent_override_level=1  view_as=Number  enum_struct={'Disabled', 'Enabled'}  use_help_units=off  parent_help=''  parent_units=''  use_min_max=off  parent_min=-inf  parent_max=inf  use_precision=off  parent_precision=''  parent_gain=1  parent_offset=0  parent_exp=1  use_mototune_group=off  parent_group=motohawk_vardec_path(gcb)
  motohawk_override_abs12 : MotoHawk_lib/Calibration & Probing Blocks/motohawk_override_abs  SystemSampleTime=-1  parent_name='Heater_Temp_Raw_Ovr'  parent_val=0  show_more=off  name_source=Use Parameter  parent_read_level=1  parent_override_level=1  view_as=Number  enum_struct={'Disabled', 'Enabled'}  use_help_units=off  parent_help=''  parent_units=''  use_min_max=off  parent_min=-inf  parent_max=inf  use_precision=off  parent_precision=''  parent_gain=1  parent_offset=0  parent_exp=1  use_mototune_group=off  parent_group=motohawk_vardec_path(gcb)
  motohawk_override_abs2 : MotoHawk_lib/Calibration & Probing Blocks/motohawk_override_abs  SystemSampleTime=-1  parent_name='Heater_Core_Blend_Valve_Ovr'  parent_val=0  show_more=off  name_source=Use Parameter  parent_read_level=1  parent_override_level=1  view_as=Number  enum_struct={'Disabled', 'Enabled'}  use_help_units=off  parent_help=''  parent_units=''  use_min_max=off  parent_min=-inf  parent_max=inf  use_precision=off  parent_precision=''  parent_gain=1  parent_offset=0  parent_exp=1  use_mototune_group=off  parent_group=motohawk_vardec_path(gcb)
  motohawk_probe1 : MotoHawk_lib/Calibration & Probing Blocks/motohawk_probe  nam='Radiator_Blend_Valve_Probe'  show_more=off  name_source=Use Parameter  read_level=1  view_as=Number  enum_struct={'Disabled', 'Enabled'}  vector_style=Wide Row  use_help_units=off  help=''  units=''  use_header_enum=off  row_header_enum={}  col_header_enum={}  use_precision=off  precision=''  gain=1  offset=0  exp=1  use_mototune_group=off  mototune_group=motohawk_vardec_path(gcb)
  motohawk_probe12 : MotoHawk_lib/Calibration & Probing Blocks/motohawk_probe  nam='Heater_Temp_Raw_Probe'  show_more=off  name_source=Use Parameter  read_level=1  view_as=Number  enum_struct={'Disabled', 'Enabled'}  vector_style=Wide Row  use_help_units=off  help=''  units=''  use_header_enum=off  row_header_enum={}  col_header_enum={}  use_precision=off  precision=''  gain=1  offset=0  exp=1  use_mototune_group=off  mototune_group=motohawk_vardec_path(gcb)
  motohawk_probe2 : MotoHawk_lib/Calibration & Probing Blocks/motohawk_probe  nam='Heater_Core_Blend_Valve_Probe'  show_more=off  name_source=Use Parameter  read_level=1  view_as=Number  enum_struct={'Disabled', 'Enabled'}  vector_style=Wide Row  use_help_units=off  help=''  units=''  use_header_enum=off  row_header_enum={}  col_header_enum={}  use_precision=off  precision=''  gain=1  offset=0  exp=1  use_mototune_group=off  mototune_group=motohawk_vardec_path(gcb)
  motohawk_probe3 : MotoHawk_lib/Calibration & Probing Blocks/motohawk_probe  nam='Heater_Temp_Probe'  show_more=off  name_source=Use Parameter  read_level=1  view_as=Number  enum_struct={'Disabled', 'Enabled'}  vector_style=Wide Row  use_help_units=off  help=''  units=''  use_header_enum=off  row_header_enum={}  col_header_enum={}  use_precision=off  precision=''  gain=1  offset=0  exp=1  use_mototune_group=off  mototune_group=motohawk_vardec_path(gcb)
  Out1 : Outport
  wires:
  Bus Creator/1 -> Out1/1
  motohawk_ain4/1 -> motohawk_override_abs12/1, motohawk_probe12/1
  motohawk_ain2/1 -> motohawk_override_abs1/1, motohawk_probe1/1
  motohawk_ain1/1 -> motohawk_override_abs2/1, motohawk_probe2/1
  motohawk_override_abs2/1 -> Data Type Conversion/1  "Heater_Core_Blend_Position"
  motohawk_override_abs1/1 -> Data Type Conversion1/1  "Radiator_Blend_Position"
  motohawk_override_abs12/1 -> Data Type Conversion2/1  "Heater_Temp"
  Data Type Conversion/1 -> Heater Core Low Pass/1(in)  "Heater_Core_Blend_Position"
  Data Type Conversion1/1 -> Radiator Low Pass/1(in)  "Radiator_Blend_Position"
  motohawk_ain4/2 -> Terminator/1
  motohawk_ain1/2 -> Terminator2/1
  motohawk_ain2/2 -> Terminator1/1
  Data Type Conversion2/1 -> Embedded MATLAB Function/1(thermistor_reading), Bus Creator/4  "Heater_Temp_Raw"
  Embedded MATLAB Function/1(temp_reading) -> Bus Creator/1, motohawk_probe3/1
  Radiator Low Pass/1(out) -> Bus Creator/2  "Radiator_Blend_Position"
  Heater Core Low Pass/1(out) -> Bus Creator/3  "Heater_Core_Blend_Position"

== system Mooventure2016_Rev5/Foreground/Inputs/Analog Inputs/DCDC Converter ==
  Terminator : Terminator
  motohawk_ain4 : MotoHawk_lib/Analog I//O Blocks/motohawk_ain  res_name=[]  text_resource=AN22  code_resource=NONE  val_resource=-1  target=ECM-5554-112-0904-xD  resource_enum_str=(None)=-1,AN24=1,AN25=2,AN26=3,AN27=4,AN28=5,AN29=6,AN30=7,AN31=8,AN32=9,AN33=10,ECUP=11,ESTOP=12,DRVP=13,XDRP=14,XDRP_B=15,AN1=16,AN2=17,AN3=18,AN4=19,AN5=20,AN6=21,AN7=22,AN8=23,AN9=24,AN10=25,AN11=26,AN12=27,AN13=28,AN14=29,AN15=30,AN16=31,AN17=32,AN18=33,AN19=34,AN20=35,AN21=36,AN22=37,AN23=38,O2A=39,O2B=40,O2C=41,O2D=42  altref=5V Reference  typ=uint16  num_adc_bits=8  use_stat=on  use_vardec=on  nam='DCDC_Conveter'  read_level=1  write_level=1  group='I/O Pins | Inputs Config'
  motohawk_override_abs12 : MotoHawk_lib/Calibration & Probing Blocks/motohawk_override_abs  SystemSampleTime=-1  parent_name='DCDC_Status_Ovr'  parent_val=0  show_more=off  name_source=Use Parameter  parent_read_level=1  parent_override_level=1  view_as=Number  enum_struct={'Disabled', 'Enabled'}  use_help_units=off  parent_help=''  parent_units=''  use_min_max=off  parent_min=-inf  parent_max=inf  use_precision=off  parent_precision=''  parent_gain=1  parent_offset=0  parent_exp=1  use_mototune_group=off  parent_group=motohawk_vardec_path(gcb)
  motohawk_probe12 : MotoHawk_lib/Calibration & Probing Blocks/motohawk_probe  nam='DCDC_Status_Prb'  show_more=off  name_source=Use Parameter  read_level=1  view_as=Number  enum_struct={'Disabled', 'Enabled'}  vector_style=Wide Row  use_help_units=off  help=''  units=''  use_header_enum=off  row_header_enum={}  col_header_enum={}  use_precision=off  precision=''  gain=1  offset=0  exp=1  use_mototune_group=off  mototune_group=motohawk_vardec_path(gcb)
  Out1 : Outport
  wires:
  motohawk_ain4/1 -> motohawk_override_abs12/1, motohawk_probe12/1
  motohawk_ain4/2 -> Terminator/1
  motohawk_override_abs12/1 -> Out1/1  "DCDStatus"
